simulink model "l1_ridealong"  (R2026a)
settings: Solver=FixedStepDiscrete  StopTime=t_final  FixedStep=dt_sim
PreLoadFcn:
  | run('l1_init.m')
undefined symbols (not defined in the file): k
libraries: l1_blocks x7
settings Model: Creator=eduno  LastModifiedBy=eduno

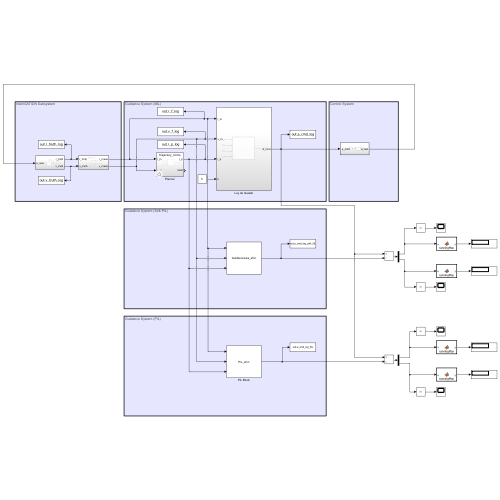
[thumbnail: Simulink's stored preview of the top-level diagram]
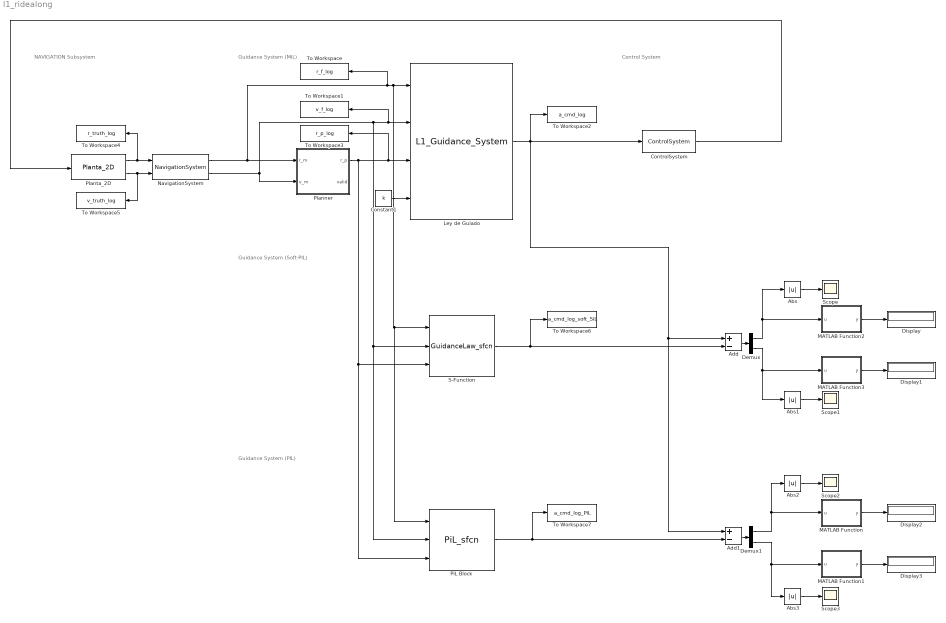
== system l1_ridealong ==
  note: Control System
  note: NAVIGATION Subsystem
  note: Guidance System (MiL)
  note: Guidance System (Soft-PIL)
  note: Guidance System (PIL)
  Abs{,1..3} (4 alike) : Abs  SaturateOnIntegerOverflow=off
  Add : Sum  Inputs=+-
  Add1 : Sum  Inputs=+-
  Constant1 : Constant  Value=k
  ControlSystem : l1_blocks/ControlSystem  SystemSampleTime=-1  VariantActivationTime=update diagram  EmptyChoice=off  PassThrough=off  PassThroughVariantControl=(default)  EmptyChoiceVariantControl=(default)  AllowFlexibleInterface=on  Latency=0  AutoFrameSizeCalculation=off
  Demux : Demux  Outputs=2
  Demux1 : Demux  Outputs=2
  Display{,1..3} (4 alike) : Display
  Ley de Guiado : l1_blocks/L1_Guidance_System  SystemSampleTime=-1  VariantActivationTime=update diagram  EmptyChoice=off  PassThrough=off  PassThroughVariantControl=(default)  EmptyChoiceVariantControl=(default)  AllowFlexibleInterface=on  Latency=0  AutoFrameSizeCalculation=off
  MATLAB Function : MATLAB Function  TreatAsAtomicUnit=on
  MATLAB Function1 : MATLAB Function  TreatAsAtomicUnit=on
  MATLAB Function2 : MATLAB Function  TreatAsAtomicUnit=on
  MATLAB Function3 : MATLAB Function  TreatAsAtomicUnit=on
  NavigationSystem : l1_blocks/NavigationSystem  SystemSampleTime=-1  VariantActivationTime=update diagram  EmptyChoice=off  PassThrough=off  PassThroughVariantControl=(default)  EmptyChoiceVariantControl=(default)  AllowFlexibleInterface=on  Latency=0  AutoFrameSizeCalculation=off
  PiL Block : S-Function  FunctionName=PiL_sfcn  SFunctionDeploymentMode=off  EnableBusSupport=off
  Planner : Subsystem  Variant=on
  Planta_2D : l1_blocks/Planta_2D  SystemSampleTime=-1  VariantActivationTime=update diagram  EmptyChoice=off  PassThrough=off  PassThroughVariantControl=(default)  EmptyChoiceVariantControl=(default)  AllowFlexibleInterface=on  Latency=0  AutoFrameSizeCalculation=off
  S-Function : S-Function  FunctionName=GuidanceLaw_sfcn  SFunctionDeploymentMode=off  EnableBusSupport=off
  Scope{,1..3} (4 alike) : Scope
      Scope settings: ActiveDisplayYMinimum=-0.00020522351922828874  ActiveDisplayYMaximum=0.0018470116730545992
      Scope1 settings: ActiveDisplayYMinimum=-1  ActiveDisplayYMaximum=1
      Scope2 settings: ActiveDisplayYMinimum=-0.00038604099091711516  ActiveDisplayYMaximum=0.0034743689182540373  DataLoggingVariableName=ScopeData2
      Scope3 settings: ActiveDisplayYMinimum=-0.000386040990917115  ActiveDisplayYMaximum=0.003474368918254036  DataLoggingVariableName=ScopeData3
  To Workspace : ToWorkspace  VariableName=r_f_log  SaveFormat=Timeseries  SampleTime=-1
  To Workspace1 : ToWorkspace  VariableName=v_f_log  SaveFormat=Timeseries  SampleTime=-1
  To Workspace2 : ToWorkspace  VariableName=a_cmd_log  SaveFormat=Timeseries  SampleTime=-1
  To Workspace3 : ToWorkspace  VariableName=r_p_log  SaveFormat=Timeseries  SampleTime=-1
  To Workspace4 : ToWorkspace  VariableName=r_truth_log  SaveFormat=Timeseries  SampleTime=-1
  To Workspace5 : ToWorkspace  VariableName=v_truth_log  SaveFormat=Timeseries  SampleTime=-1
  To Workspace6 : ToWorkspace  VariableName=a_cmd_log_soft_SiL  SaveFormat=Timeseries  SampleTime=-1
  To Workspace7 : ToWorkspace  VariableName=a_cmd_log_PiL  SaveFormat=Timeseries  SampleTime=-1
  wires:
  NavigationSystem/1 -> To Workspace/1, PiL Block/1, S-Function/1, Ley de Guiado/1, Planner/1(r_m)
  NavigationSystem/2 -> Planner/2(v_m), Ley de Guiado/2, To Workspace1/1, PiL Block/2, S-Function/2
  Constant1/1 -> Ley de Guiado/4
  Ley de Guiado/1 -> ControlSystem/1, Add1/1, Add/1, To Workspace2/1
  Planner/1(r_p) -> Ley de Guiado/3, To Workspace3/1, PiL Block/3, S-Function/3
  ControlSystem/1 -> Planta_2D/1
  Planta_2D/1 -> To Workspace4/1, NavigationSystem/1
  Planta_2D/2 -> To Workspace5/1, NavigationSystem/2
  S-Function/1 -> To Workspace6/1, Add/2
  Add/1 -> Demux/1
  Demux/1 -> MATLAB Function2/1(u), Abs/1
  Demux/2 -> MATLAB Function3/1(u), Abs1/1
  MATLAB Function2/1(y) -> Display/1
  MATLAB Function3/1(y) -> Display1/1
  Add1/1 -> Demux1/1
  Demux1/2 -> Abs3/1, MATLAB Function1/1(u)
  Demux1/1 -> MATLAB Function/1(u), Abs2/1
  PiL Block/1 -> To Workspace7/1, Add1/2
  MATLAB Function/1(y) -> Display2/1
  MATLAB Function1/1(y) -> Display3/1
  Abs/1 -> Scope/1
  Abs1/1 -> Scope1/1
  Abs2/1 -> Scope2/1
  Abs3/1 -> Scope3/1

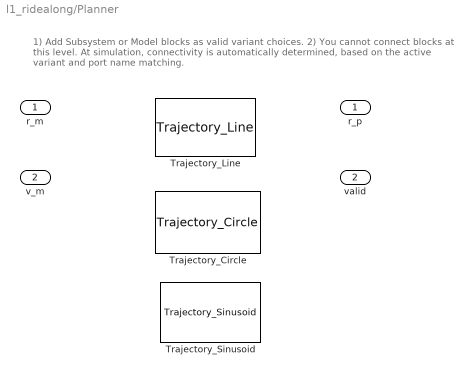
== system l1_ridealong/Planner ==
  note: 1) Add Subsystem or Model blocks as valid variant choices.
      | 2) You cannot connect blocks at this level. At simulation, connectivity is automatically
      | determined, based on the active variant and port name matching.
  r_m : Inport
  v_m : Inport  Port=2
  Trajectory_Circle : l1_blocks/Trajectory_Circle  SystemSampleTime=-1  VariantControl=VAR_CIRCLE  VariantActivationTime=update diagram  EmptyChoice=off  PassThrough=off  PassThroughVariantControl=(default)  EmptyChoiceVariantControl=(default)  AllowFlexibleInterface=on  Latency=0  AutoFrameSizeCalculation=off
  Trajectory_Line : l1_blocks/Trajectory_Line  SystemSampleTime=-1  VariantControl=VAR_LINE  VariantActivationTime=update diagram  EmptyChoice=off  PassThrough=off  PassThroughVariantControl=(default)  EmptyChoiceVariantControl=(default)  AllowFlexibleInterface=on  Latency=0  AutoFrameSizeCalculation=off
  Trajectory_Sinusoid : l1_blocks/Trajectory_Sinusoid  SystemSampleTime=-1  VariantControl=VAR_SINUSOID  VariantActivationTime=update diagram  EmptyChoice=off  PassThrough=off  PassThroughVariantControl=(default)  EmptyChoiceVariantControl=(default)  AllowFlexibleInterface=on  Latency=0  AutoFrameSizeCalculation=off
  r_p : Outport
  valid : Outport  Port=2

== matlab function l1_ridealong/MATLAB Function ==
  data: u input; y output
function y = runningMax(u)
persistent maxVal3

if isempty(maxVal3)
    maxVal3 = abs(u);
elseif u > maxVal3
    maxVal3 = abs(u);
end

y = maxVal3;
end

== matlab function l1_ridealong/MATLAB Function2 ==
  data: u input; y output
function y = runningMax(u)
persistent maxVal1

if isempty(maxVal1)
    maxVal1 = abs(u);
elseif u > maxVal1
    maxVal1 = abs(u);
end

y = maxVal1;
end

== matlab function l1_ridealong/MATLAB Function3 ==
  data: u input; y output
function y = runningMax(u)
persistent maxVal2

if isempty(maxVal2)
    maxVal2 = abs(u);
elseif u > maxVal2
    maxVal2 = abs(u);
end

y = maxVal2;
end

== matlab function l1_ridealong/MATLAB Function1 ==
  data: u input; y output
function y = runningMax(u)
persistent maxVal4

if isempty(maxVal4)
    maxVal4 = abs(u);
elseif u > maxVal4
    maxVal4 = abs(u);
end

y = maxVal4;
end
